simulink model "counter_Timer"  (R2023b)
settings: Solver=FixedStepAuto  StartTime=0.0  StopTime=inf  FixedStep=1  RelTol=1e-3
libraries: simulink x1
settings Model: Creator=Beshary  LastModifiedBy=Beshary
settings OptimizationCC: DefaultParameterBehavior=Inlined  EnhancedBackFolding=on  PassReuseOutputArgsAs=Individual arguments  ZeroExternalMemoryAtStartup=off  ZeroInternalMemoryAtStartup=off  OptimizeBlockOrder=speed  DifferentSizesBufferReuse=on  OptimizationCustomize=off  EfficientTunableParamExpr=on
settings DebuggingCC: ParameterTunabilityLossMsg=error
settings SFSimCC: MATLABDynamicMemAlloc=off
settings RTWCC: Description=Embedded Coder  SystemTargetFile=ert.tlc  TemplateMakefile=ert_default_tmf
settings CodeAppCC: ForceParamTrailComments=on  IgnoreCustomStorageClasses=off  OperatorAnnotations=on  SimulinkDataObjDesc=on  SFDataObjDesc=on  InsertBlockDesc=on
settings ERTTargetCC: TargetLangStandard=C99 (ISO)  GenerateSampleERTMain=on  InlinedParameterPlacement=NonHierarchical  ERTCustomFileTemplate=example_file_process.tlc

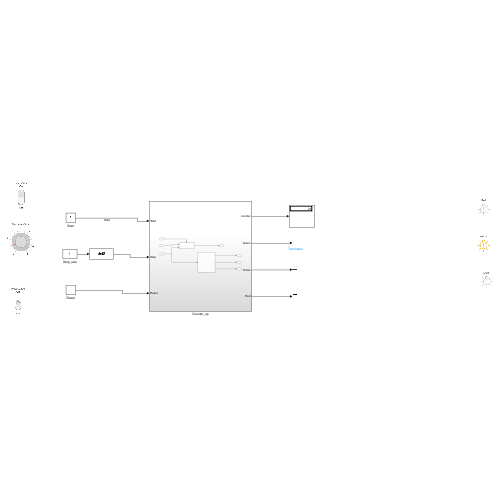
[thumbnail: Simulink's stored preview of the top-level diagram]
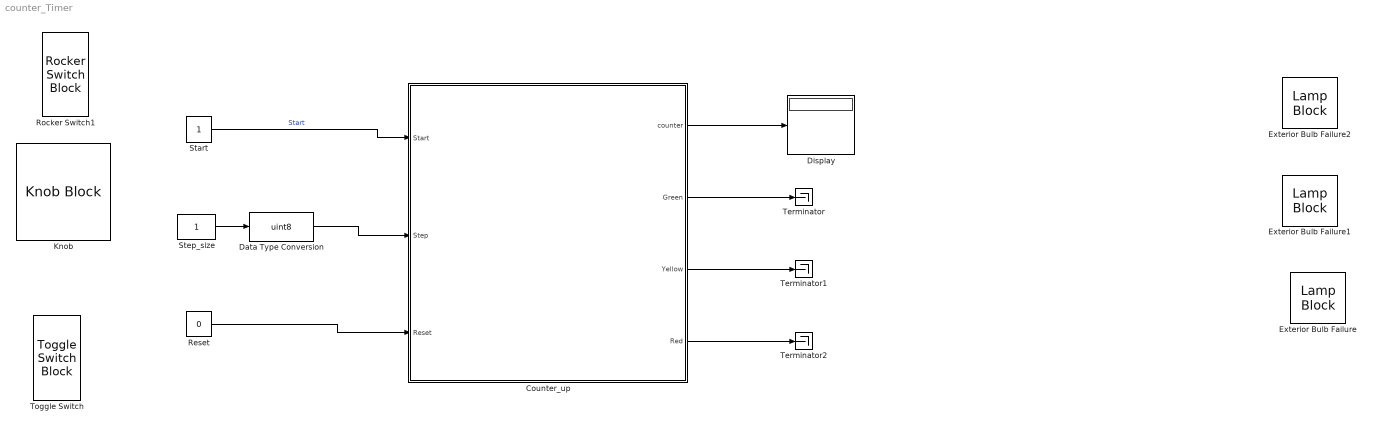
== system counter_Timer ==
  Counter_up : Subsystem
  Data Type Conversion : DataTypeConversion  OutDataTypeStr=uint8  SaturateOnIntegerOverflow=off  RndMeth=Floor
  Display : Display
  Exterior Bulb Failure : LampBlock  Icon=ExteriorBulbFailure
  Exterior Bulb Failure1 : LampBlock  Icon=ExteriorBulbFailure
  Exterior Bulb Failure2 : LampBlock  Icon=ExteriorBulbFailure
  Knob : KnobBlock  ScaleMax=8  TickInterval=1
  Reset : Constant  Value=0
  Rocker Switch1 : RockerSwitchBlock
      settings: Values={{'Off', 'On'}, [0 1]}
  Start : Constant  OutDataTypeStr=boolean
  Step_size : Constant  OutDataTypeStr=int8
  Terminator : Terminator
  Terminator1 : Terminator
  Terminator2 : Terminator
  Toggle Switch : ToggleSwitchBlock
      settings: Values={{'Off', 'On'}, [0 1]}
  wires:
  Start/1 -> Counter_up/1(Start)  "Start"
  Step_size/1 -> Data Type Conversion/1
  Reset/1 -> Counter_up/3(Reset)
  Counter_up/1(counter) -> Display/1
  Data Type Conversion/1 -> Counter_up/2(Step)
  Counter_up/4(Red) -> Terminator2/1
  Counter_up/3(Yellow) -> Terminator1/1
  Counter_up/2(Green) -> Terminator/1

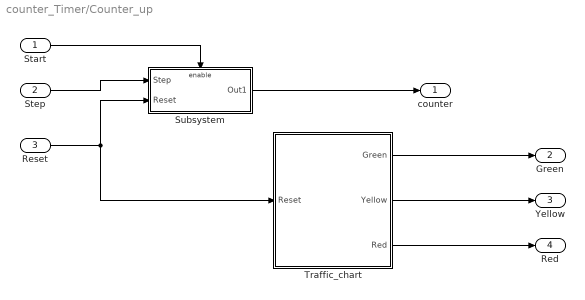
== system counter_Timer/Counter_up ==
  Start : Inport
  Step : Inport  Port=2
  Reset : Inport  Port=3
  Subsystem : Subsystem
  Traffic_chart : Subsystem
  counter : Outport
  Green : Outport  Port=2
  Yellow : Outport  Port=3
  Red : Outport  Port=4
  wires:
  Step/1 -> Subsystem/1(Step)
  Start/1 -> Subsystem/Enable
  Subsystem/1(Out1) -> counter/1
  Reset/1 -> Subsystem/2(Reset), Traffic_chart/1(Reset)
  Traffic_chart/3(Red) -> Red/1
  Traffic_chart/1(Green) -> Green/1
  Traffic_chart/2(Yellow) -> Yellow/1

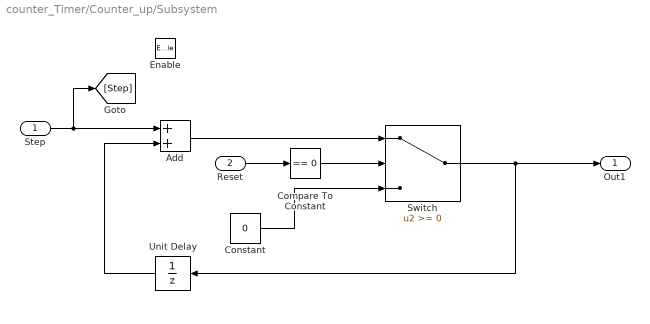
== system counter_Timer/Counter_up/Subsystem ==
  Step : Inport
  Reset : Inport  Port=2
  Enable : EnablePort
  Add : Sum
  Compare To Constant : simulink/Logic and Bit Operations/Compare To Constant  relop===  const=0  OutDataTypeStr=boolean
  Constant : Constant  Value=0
  Switch : Switch  SaturateOnIntegerOverflow=off  InputSameDT=off
  Unit Delay : UnitDelay  SampleTime=-1  HasFrameUpgradeWarning=on
  Out1 : Outport
  wires:
  Step/1 -> [Step], Add/1
  Unit Delay/1 -> Add/2
  Switch/1 -> Unit Delay/1, Out1/1
  Reset/1 -> Compare To Constant/1
  Add/1 -> Switch/1
  Constant/1 -> Switch/3
  Compare To Constant/1 -> Switch/2

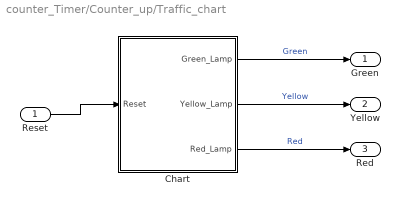
== system counter_Timer/Counter_up/Traffic_chart ==
  Reset : Inport
  Chart : Stateflow chart  TreatAsAtomicUnit=on
  Green : Outport
  Yellow : Outport  Port=2
  Red : Outport  Port=3
  wires:
  Chart/1(Green_Lamp) -> Green/1  "Green"
  Chart/3(Red_Lamp) -> Red/1  "Red"
  Chart/2(Yellow_Lamp) -> Yellow/1  "Yellow"
  Reset/1 -> Chart/1(Reset)

== stateflow chart counter_Timer/Counter_up/Traffic_chart/Chart ==
  state Yellow
    en:
    Yellow_Lamp=1;
    ex:
    Yellow_Lamp=0;
    support_transtion=1;
  state Green
    en:
    Green_Lamp=1;
    ex:
    Green_Lamp=0;
    support_transtion=0;
  state Red
    en:
    Red_Lamp=1;
    ex:
    Red_Lamp=0;
  Green -> Red [order 1] : [Reset==1]
  Yellow -> Red [order 1] : [Reset==1]{support_transtion=1}
  (default) -> Red
  Red -> Yellow : [after(8,sec)]
  Yellow -> Green [order 3] : [after(5,sec)&&support_transtion==1]
  Yellow -> Red [order 2] : [after(5,sec)&&support_transtion==0]
  Green -> Yellow [order 2] : [after(8,sec)&&support_transtion==1]
  data: Green_Lamp output; Yellow_Lamp output; Red_Lamp output; support_transtion local =1; Reset input
